simulink model "untitled"  (R2019a)
settings: Solver=VariableStepAuto  StartTime=0.0  StopTime=10.0  RelTol=1e-3
settings Model: Creator=anton  LastModifiedBy=anton

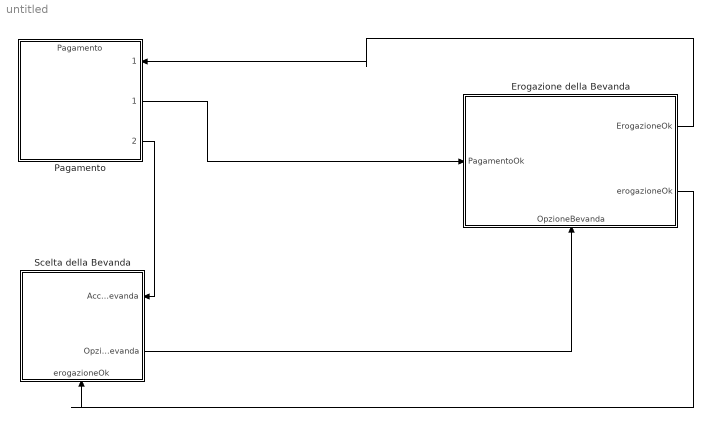
== system untitled ==
  Erogazione della Bevanda : Subsystem
      settings: PortSchema="{\"entries\":[{\"content\":{\"headerSize\":26,\"margin\":15,\"minimumSpacing\":25,\"sides\":[{\"content\":{\"connectorIds\":[\"In1\"]},\"type\":\"ConnectorPlacement.EquallySpacedRectSide\",\"uuid\":\"9001291f-2c01-497d-b978-c9da1a5dfe2f\"},{\"content\":{\"connectorIds\":[\"Out1\",\"Out2\"],\"side\":\"RIGHT\"},\"type\":\"ConnectorPlacement.EquallySpacedRectSide\",\"uuid\":\"e239534c-f548-484c-979d-c6062b0b6a09\"},{\"content\":{\"connectorIds\":[],\"side\":\"TOP\"},\"type\":\"ConnectorPlacement.EquallySpacedRectSide\",\"uuid\":\"b9e248ae-18f1-4713-ac0e-a2227ceb5e9f\"},{\"content\":{\"connectorIds\":[\"In2\"],\"side\":\"BOTTOM\"},\"type\":\"ConnectorPlacement.EquallySpacedRectSide\",\"uuid\":\"569884a8-bd8b-4a35-b514-adcb73c551fa\"}]},\"type\":\"ConnectorPlacement.EquallySpacedConnector\",\"uuid\":\"dbeef95e-7cef-48b9-bf12-ea66c4821a3c\"}],\"packageUris\":[\"http:\\/\\/schema.mathworks.com\\/mf0\\/Connector\\/19700101\"],\"version\":\"1.0\"}"
  Pagamento : ModelReference  ModelNameDialog=Pagamento  SimulationMode=Normal  ModelReferenceVersion=1.1
      settings: PortSchema="{\"entries\":[{\"content\":{\"headerSize\":38,\"margin\":15,\"minimumSpacing\":25,\"sides\":[{\"content\":{\"connectorIds\":[]},\"type\":\"ConnectorPlacement.EquallySpacedRectSide\",\"uuid\":\"9001291f-2c01-497d-b978-c9da1a5dfe2f\"},{\"content\":{\"connectorIds\":[\"In1\",\"Out1\",\"Out2\"],\"side\":\"RIGHT\"},\"type\":\"ConnectorPlacement.EquallySpacedRectSide\",\"uuid\":\"e239534c-f548-484c-979d-c6062b0b6a09\"},{\"content\":{\"connectorIds\":[],\"side\":\"TOP\"},\"type\":\"ConnectorPlacement.EquallySpacedRectSide\",\"uuid\":\"b9e248ae-18f1-4713-ac0e-a2227ceb5e9f\"}]},\"type\":\"ConnectorPlacement.EquallySpacedConnector\",\"uuid\":\"dbeef95e-7cef-48b9-bf12-ea66c4821a3c\"}],\"packageUris\":[\"http:\\/\\/schema.mathworks.com\\/mf0\\/Connector\\/19700101\"],\"version\":\"1.0\"}"
  Scelta della Bevanda : Subsystem
      settings: PortSchema="{\"entries\":[{\"content\":{\"headerSize\":26,\"margin\":15,\"minimumSpacing\":25,\"sides\":[{\"content\":{\"connectorIds\":[]},\"type\":\"ConnectorPlacement.EquallySpacedRectSide\",\"uuid\":\"9001291f-2c01-497d-b978-c9da1a5dfe2f\"},{\"content\":{\"connectorIds\":[\"In2\",\"Out1\"],\"side\":\"RIGHT\"},\"type\":\"ConnectorPlacement.EquallySpacedRectSide\",\"uuid\":\"e239534c-f548-484c-979d-c6062b0b6a09\"},{\"content\":{\"connectorIds\":[],\"side\":\"TOP\"},\"type\":\"ConnectorPlacement.EquallySpacedRectSide\",\"uuid\":\"b9e248ae-18f1-4713-ac0e-a2227ceb5e9f\"},{\"content\":{\"connectorIds\":[\"In1\"],\"side\":\"BOTTOM\"},\"type\":\"ConnectorPlacement.EquallySpacedRectSide\",\"uuid\":\"1239d1ee-68d1-4a36-9de5-7c855f25f77a\"}]},\"type\":\"ConnectorPlacement.EquallySpacedConnector\",\"uuid\":\"dbeef95e-7cef-48b9-bf12-ea66c4821a3c\"}],\"packageUris\":[\"http:\\/\\/schema.mathworks.com\\/mf0\\/Connector\\/19700101\"],\"version\":\"1.0\"}"
  wires:
  Scelta della Bevanda/1(OpzioneBevanda) -> Erogazione della Bevanda/2(OpzioneBevanda)
  Erogazione della Bevanda/2(erogazioneOk) -> Scelta della Bevanda/1(erogazioneOk)
  Erogazione della Bevanda/1(ErogazioneOk) -> Pagamento/1
  Pagamento/2 -> Scelta della Bevanda/2(Accetta Bevanda)
  Pagamento/1 -> Erogazione della Bevanda/1(PagamentoOk)

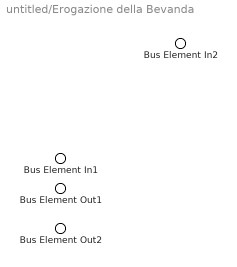
== system untitled/Erogazione della Bevanda ==
  Bus Element In2 : Inport  PortName=PagamentoOk
  Bus Element In1 : Inport  Port=2  PortName=OpzioneBevanda
  Bus Element Out1 : Outport  PortName=ErogazioneOk
  Bus Element Out2 : Outport  Port=2  PortName=erogazioneOk

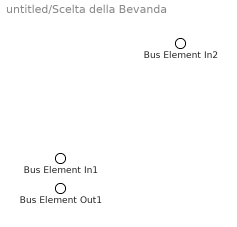
== system untitled/Scelta della Bevanda ==
  Bus Element In2 : Inport  PortName=erogazioneOk
  Bus Element In1 : Inport  Port=2  PortName=Accetta Bevanda
  Bus Element Out1 : Outport  PortName=OpzioneBevanda
